simulink model "Gait_EKF"  (R2025b)
settings: Solver=FixedStepAuto  StartTime=0.0  StopTime=1.175  FixedStep=1e-3  RelTol=1e-3
values from neighbouring files (symbols this model uses):
  Phase = [0 0.087266463 0.174532925 0.261799388 0.34906585 0.436332313 0.523598776 0.610865238 0.698131701 0.785398163 0.872664626 0.959931089 ... (73 elements, 73x1)]    [Data.mat]    (also in ankle_velocity.mat)
  phaseDot = [5.2359867328 5.2359882736 5.2359882736 5.2359867028 5.2359882736 5.2359883036 5.2359867028 5.2359882736 5.2359882736 5.2359867028 5.2359883036 5.2359882736 ... (73 elements, 73x1)]    [Data.mat]    (also in ankle_velocity.mat)
settings Model: Creator=ouka1  LastModifiedBy=ouka1

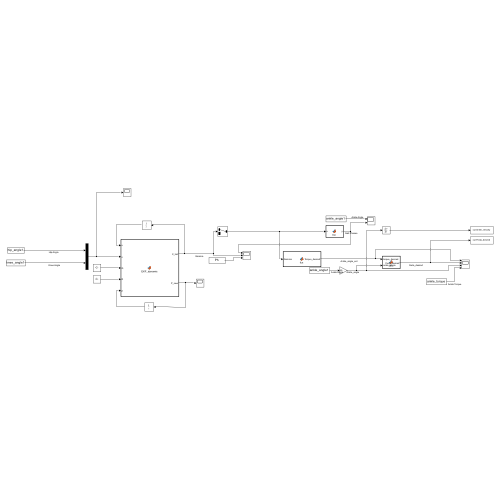
[thumbnail: Simulink's stored preview of the top-level diagram]
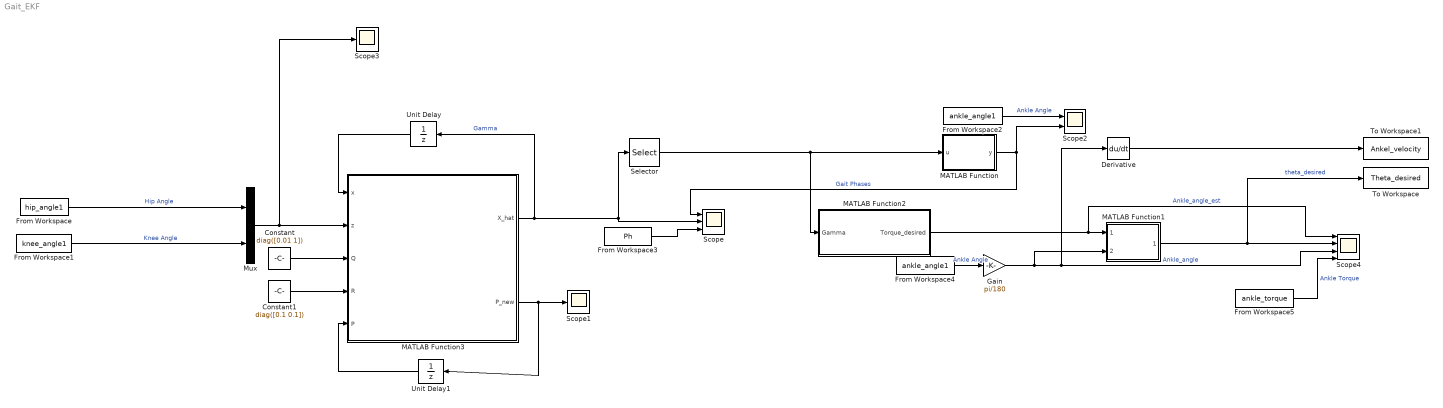
== system Gait_EKF ==
  Constant : Constant  Value=diag([0.01 1])
  Constant1 : Constant  Value=diag([0.1 0.1])
  Derivative : Derivative
  From Workspace : FromWorkspace  VariableName=hip_angle1
  From Workspace1 : FromWorkspace  VariableName=knee_angle1
  From Workspace2 : FromWorkspace  VariableName=ankle_angle1
  From Workspace3 : FromWorkspace  VariableName=Ph
  From Workspace4 : FromWorkspace  VariableName=ankle_angle1
  From Workspace5 : FromWorkspace  VariableName=ankle_torque
  Gain : Gain  Gain=pi/180
  MATLAB Function : MATLAB Function  TreatAsAtomicUnit=on
  MATLAB Function1 : MATLAB Function  TreatAsAtomicUnit=on
  MATLAB Function2 : MATLAB Function  TreatAsAtomicUnit=on
  MATLAB Function3 : MATLAB Function  TreatAsAtomicUnit=on
  Mux : Mux  Inputs=2
  Scope : Scope  NumInputPorts=3
      settings: ActiveDisplayYMinimum=-1.0455946681093786  ActiveDisplayYMaximum=9.0050660742343762
  Scope1 : Scope
      settings: ActiveDisplayYMinimum=-0.819736933959527  ActiveDisplayYMaximum=7.3776324056357447
  Scope2 : Scope  NumInputPorts=2
      settings: ActiveDisplayYMinimum=-1  ActiveDisplayYMaximum=1  DataLoggingVariableName=ScopeData2
  Scope3 : Scope
      settings: ActiveDisplayYMinimum=-80.871706567823807  ActiveDisplayYMaximum=32.795184662620741  DataLoggingVariableName=ScopeData3
  Scope4 : Scope  NumInputPorts=4
      settings: ActiveDisplayYMinimum=-0.656612633550641  ActiveDisplayYMaximum=3.0827219552173637  DataLoggingVariableName=ScopeData4
  Selector : Selector  InputPortWidth=2  IndexOptions=Index vector (dialog)  Indices=[1]  OutputSizes=1
  To Workspace : ToWorkspace  VariableName=Theta_desired  SaveFormat=Timeseries  SampleTime=-1
  To Workspace1 : ToWorkspace  VariableName=Ankel_velocity  SaveFormat=Timeseries  SampleTime=-1
  Unit Delay : UnitDelay  InitialCondition=[Phase(2); phaseDot(2)]  SampleTime=-1  HasFrameUpgradeWarning=on
  Unit Delay1 : UnitDelay  InitialCondition=zeros(2,2)  SampleTime=-1  HasFrameUpgradeWarning=on
  wires:
  From Workspace/1 -> Mux/1  "Hip Angle"
  From Workspace1/1 -> Mux/2  "Knee Angle"
  From Workspace2/1 -> Scope2/1  "Ankle Angle"
  Mux/1 -> Scope3/1, MATLAB Function3/2(z)
  Constant/1 -> MATLAB Function3/3(Q)
  Constant1/1 -> MATLAB Function3/4(R)
  MATLAB Function3/2(P_new) -> Scope1/1, Unit Delay1/1
  MATLAB Function3/1(X_hat) -> Unit Delay/1, Selector/1, Scope/2  "Gamma"
  Unit Delay/1 -> MATLAB Function3/1(x)
  Unit Delay1/1 -> MATLAB Function3/5(P)
  From Workspace3/1 -> Scope/3
  MATLAB Function/1(y) -> Scope2/2, Scope/1  "Gait Phases"
  Selector/1 -> MATLAB Function2/1(Gamma), MATLAB Function/1(u)
  MATLAB Function2/1(Torque_desired) -> Scope4/1, MATLAB Function1/1(torque_desired)  "Ankle_angle_est"
  MATLAB Function1/1(theta_desired) -> To Workspace/1, Scope4/2  "theta_desired"
  From Workspace4/1 -> Gain/1  "Ankle Angle"
  From Workspace5/1 -> Scope4/4  "Ankle Torque"
  Gain/1 -> Derivative/1, Scope4/3, MATLAB Function1/2(ankle_angle)  "Ankle_angle"
  Derivative/1 -> To Workspace1/1

== matlab function Gait_EKF/MATLAB Function1 ==
  data: torque_desired input; theta_desired output; ankle_angle input; K_opt parameter
function theta_desired = fcn(torque_desired,ankle_angle,K_opt)
theta_desired = -(torque_desired/K_opt) + ankle_angle;
end

== matlab function Gait_EKF/MATLAB Function ==
  data: u input; y output
function y = fcn(u)
    if u <= 0
        y = 1;
    elseif u <= 0.610865238
        y = 1;
    elseif u <= 1.221730476
        y = 2;
    elseif u <= 2.443460953
        y = 3;
    elseif u <= 3.490658504
        y = 4;
    elseif u <= 4.276056667
        y = 5;
    elseif u <= 4.625122518
        y = 6;
    elseif u <= 5.672320069
        y = 7;
    else
        y = 8;
    end
end

== matlab function Gait_EKF/MATLAB Function2 ==
  data: Gamma input; Torque_desired output
function Torque_desired = fcn(Gamma)
x=Gamma;
a0  = -30.996;
a1  =  43.013;    
b1  =   -30.54;  
a2  = -10.643;  
b2  =   22.996;   
a3  =   8.4676;   
b3  =  -3.5524;   
a4  =  -8.5763;   
b4  =    4.451;     
a5  =   4.9492;     
b5  =  0.8472;   
a6  =   -3.999;   
b6  =   0.4491;    
w   =   0.9332;    
Torque_desired = a0 + a1*cos(x*w) + b1*sin(x*w) + a2*cos(2*x*w) + b2*sin(2*x*w) + a3*cos(3*x*w) + b3*sin(3*x*w) + a4*cos(4*x*w) + b4*sin(4*x*w) + a5*cos(5*x*w) + b5*sin(5*x*w) + a6*cos(6*x*w) + b6*sin(6*x*w);


end

== matlab function Gait_EKF/MATLAB Function3 ==
  data: x input size=[2 1]; X_hat output size=[2 1]; z input; Q input; R input; P input; P_new output; dt parameter
function [X_hat, P_new] = EKF_dynamic(x, z, Q, R, P, dt)

%% 1. Prediction Step
    F = [1, dt; 
         0, 1];
         
    X_prior = F * x;
    if X_prior(1) >= 2*pi
        X_prior(1) = 0;
    end
    P_prior = F * P * F' + Q;

    % Extract the predicted phase to use for non-linear evaluations
    Gamma = X_prior(1); 

%% 2. Evaluate Non-Linear Measurement Equations (z_pred)
    % Hip Angle (Theta) - 2nd Order Fourier, w = 1.1916
    Theta_pred = 0.4012 + 17.969*cos(Gamma*1.1916) + 10.652*sin(Gamma*1.1916)...
                 + 1.9287*cos(2*Gamma*1.1916) - 1.6561*sin(2*Gamma*1.1916);

    % Knee Angle (Phi) - 3rd Order Fourier, w = 0.9437
    Phi_pred = -22.906 + 6.1848*cos(Gamma*0.9437) + 18.761*sin(Gamma*0.9437)...
               + 15.975*cos(2*Gamma*0.9437) - 15.451*sin(2*Gamma*0.9437)...
               - 3.2965*cos(3*Gamma*0.9437) - 6.6207*sin(3*Gamma*0.9437);

    % Ankle Angle (Alpha) - 5th Order Fourier, w = 0.9958
    % Alpha_pred = 3.7427 - 4.8038*cos(Gamma*0.9958) + 3.3752*sin(Gamma*0.9958)...
    %              + 2.3591*cos(2*Gamma*0.9958) - 2.4098*sin(2*Gamma*0.9958)...
    %              - 3.0979*cos(3*Gamma*0.9958) - 1.4657*sin(3*Gamma*0.9958)...
    %              + 0.9641*cos(4*Gamma*0.9958) + 1.6091*sin(4*Gamma*0.9958)...
    %              + 1.1655*cos(5*Gamma*0.9958) - 1.4288*sin(5*Gamma*0.9958);

    % Combine into the predicted measurement vector
    z_pred = [Theta_pred; Phi_pred];

%% 3. Evaluate the Jacobian (H) at the Predicted State
    % Hip Angle Derivative (w = 1.1916)
    dTheta_dGamma = -17.969 * (1 * 1.1916) * sin(Gamma * 1.1916) ...
                    + 10.652 * (1 * 1.1916) * cos(Gamma * 1.1916) ...
                    - 1.9287 * (2 * 1.1916) * sin(2 * Gamma * 1.1916) ...
                    - 1.6561 * (2 * 1.1916) * cos(2 * Gamma * 1.1916);
    
    % Knee Angle Derivative (w = 0.9437)
    dPhi_dGamma = -6.1848 * (1 * 0.9437) * sin(Gamma * 0.9437) ...
                  + 18.761 * (1 * 0.9437) * cos(Gamma * 0.9437) ...
                  - 15.975 * (2 * 0.9437) * sin(2 * Gamma * 0.9437) ...
                  - 15.451 * (2 * 0.9437) * cos(2 * Gamma * 0.9437) ...
                  - (-3.2965) * (3 * 0.9437) * sin(3 * Gamma * 0.9437) ...
                  - 6.6207 * (3 * 0.9437) * cos(3 * Gamma * 0.9437);
    
    % Ankle Angle Derivative (w = 0.9958)
    dAlpha_dGamma = -(-4.8038) * (1 * 0.9958) * sin(Gamma * 0.9958) ...
                    + 3.3752 * (1 * 0.9958) * cos(Gamma * 0.9958) ...
                    - 2.3591 * (2 * 0.9958) * sin(2 * Gamma * 0.9958) ...
                    - 2.4098 * (2 * 0.9958) * cos(2 * Gamma * 0.9958) ...
                    - (-3.0979) * (3 * 0.9958) * sin(3 * Gamma * 0.9958) ...
                    - 1.4657 * (3 * 0.9958) * cos(3 * Gamma * 0.9958) ...
                    - 0.9641 * (4 * 0.9958) * sin(4 * Gamma * 0.9958) ...
                    + 1.6091 * (4 * 0.9958) * cos(4 * Gamma * 0.9958) ...
                    - 1.1655 * (5 * 0.9958) * sin(5 * Gamma * 0.9958) ...
                    - 1.4288 * (5 * 0.9958) * cos(5 * Gamma * 0.9958);

    % Construct the 3x2 Jacobian matrix
    H = [dTheta_dGamma, 0;
         dPhi_dGamma,   0];

%% 4. Innovation & Update Step
    % Calculate Residual
    r = z - z_pred; 
    
    % Innovation Covariance
    S = H * P_prior * H' + R;
    
    % Kalman Gain
    K = P_prior * H' / S; 
    
    % State and Covariance Update
    I = eye(2);
    P_new = (I - K * H) * P_prior * (I - K * H)' + K * R * K'; % Joseph form
    X_hat = X_prior + K * r;
    
end
